simulink model "w1p3"  (R2020a)
settings: Solver=VariableStepAuto  StartTime=0.0  StopTime=0.1  RelTol=1e-3
settings Model: Creator=Shubham  LastModifiedBy=Shubham

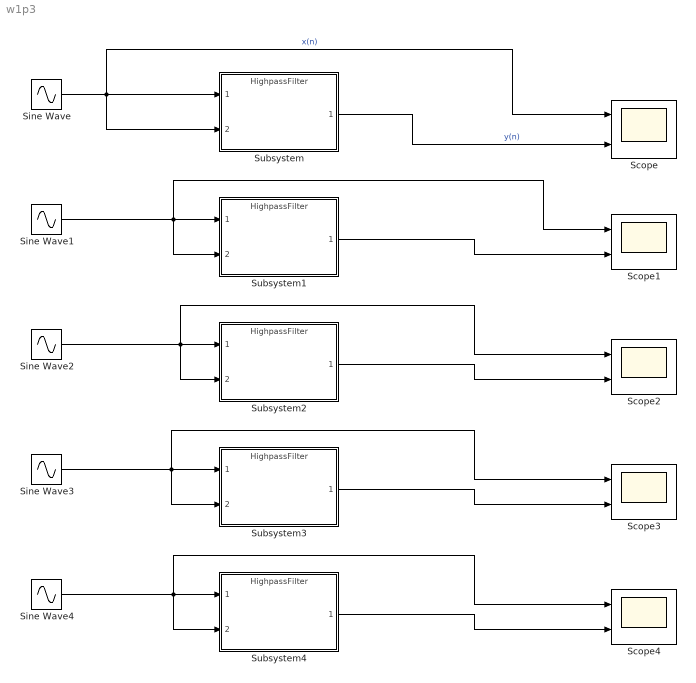
== system w1p3 ==
  Scope{,1..4} (5 alike) : Scope  NumInputPorts=2
  Sine Wave : Sin  Frequency=6280  SampleTime=0
  Sine Wave1 : Sin  Frequency=628  SampleTime=0
  Sine Wave2 : Sin  SampleTime=0
  Sine Wave3 : Sin  SampleTime=0
  Sine Wave4 : Sin  SampleTime=0
  Subsystem{,1..4} (5 alike) : ModelReference  ModelNameDialog=HighpassFilter  SimulationMode=Normal  ModelReferenceVersion=1.4
  wires:
  Sine Wave/1 -> Scope/1, Subsystem/2, Subsystem/1  "x(n)"
  Subsystem/1 -> Scope/2  "y(n)"
  Sine Wave4/1 -> Subsystem4/2, Scope4/1, Subsystem4/1
  Sine Wave3/1 -> Scope3/1, Subsystem3/2, Subsystem3/1
  Sine Wave2/1 -> Scope2/1, Subsystem2/2, Subsystem2/1
  Sine Wave1/1 -> Scope1/1, Subsystem1/2, Subsystem1/1
  Subsystem1/1 -> Scope1/2
  Subsystem2/1 -> Scope2/2
  Subsystem3/1 -> Scope3/2
  Subsystem4/1 -> Scope4/2
